simulink model "Practica7"  (R2020b)
settings: Solver=VariableStepAuto  StartTime=0.0  StopTime=20  RelTol=1e-3
settings Model: Creator=diego  LastModifiedBy=diego

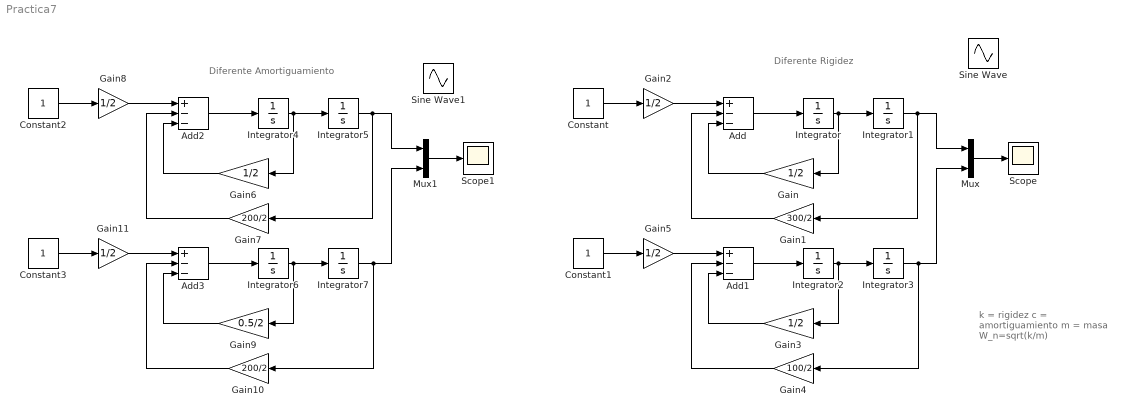
== system Practica7 ==
  note: k = rigidez
      | c = amortiguamiento
      | m = masa
      |
      | W_n=sqrt(k/m)
  note: Diferente Rigidez
  note: Diferente Amortiguamiento
  Add{,1..3} (4 alike) : Sum  Inputs=+--
  Constant{,1..3} (4 alike) : Constant
  Gain{,2..3,5..6,8,11} (7 alike) : Gain  Gain=1/2
  Gain1 : Gain  Gain=300/2
  Gain10 : Gain  Gain=200/2
  Gain4 : Gain  Gain=100/2
  Gain7 : Gain  Gain=200/2
  Gain9 : Gain  Gain=0.5/2
  Integrator{,2,4,6} (4 alike) : Integrator
  Integrator{1,3,5,7} (4 alike) : Integrator  InitialCondition=1
  Mux : Mux  Inputs=2
  Mux1 : Mux  Inputs=2
  Scope : Scope
  Scope1 : Scope
  Sine Wave : Sin  Frequency=3*2*pi  SampleTime=0.0001
  Sine Wave1 : Sin  Frequency=10*2*pi  SampleTime=0.0001
  wires:
  Integrator/1 -> Gain/1, Integrator1/1
  Add/1 -> Integrator/1
  Gain1/1 -> Add/2
  Gain/1 -> Add/3
  Constant/1 -> Gain2/1
  Gain2/1 -> Add/1
  Mux/1 -> Scope/1
  Integrator1/1 -> Gain1/1, Mux/1
  Integrator2/1 -> Gain3/1, Integrator3/1
  Gain5/1 -> Add1/1
  Constant1/1 -> Gain5/1
  Gain3/1 -> Add1/3
  Gain4/1 -> Add1/2
  Add1/1 -> Integrator2/1
  Integrator3/1 -> Gain4/1, Mux/2
  Integrator7/1 -> Gain10/1, Mux1/2
  Gain10/1 -> Add3/2
  Constant3/1 -> Gain11/1
  Gain9/1 -> Add3/3
  Gain11/1 -> Add3/1
  Integrator6/1 -> Gain9/1, Integrator7/1
  Mux1/1 -> Scope1/1
  Integrator4/1 -> Gain6/1, Integrator5/1
  Gain8/1 -> Add2/1
  Constant2/1 -> Gain8/1
  Gain6/1 -> Add2/3
  Gain7/1 -> Add2/2
  Add2/1 -> Integrator4/1
  Add3/1 -> Integrator6/1
  Integrator5/1 -> Gain7/1, Mux1/1
